simulink model "evaporator_test"  (R2019a)
settings: Solver=VariableStepAuto  StartTime=0.0  StopTime=5000*4  RelTol=1e-3
settings Model: Creator=amah2  LastModifiedBy=kovim

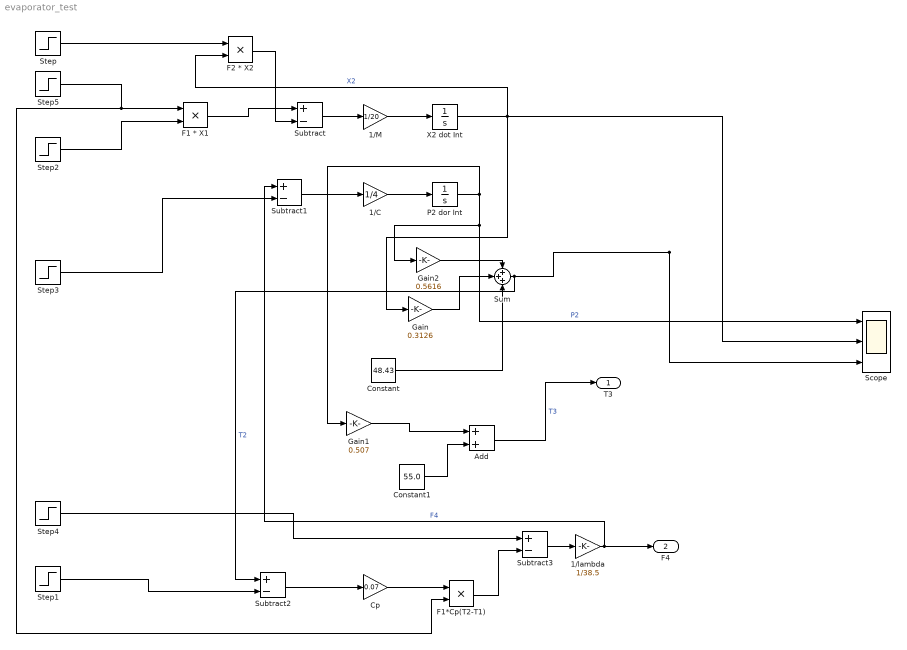
== system evaporator_test ==
  1/C : Gain  Gain=1/4
  1/M : Gain  Gain=1/20
  1/lambda : Gain  Gain=1/38.5
  Add : Sum
  Constant : Constant  Value=48.43
  Constant1 : Constant  Value=55.0
  Cp : Gain  Gain=0.07
  F1 * X1 : Product
  F1*Cp(T2-T1) : Product
  F2 * X2 : Product
  Gain : Gain  Gain=0.3126
  Gain1 : Gain  Gain=0.507
  Gain2 : Gain  Gain=0.5616
  P2 dor Int : Integrator  InitialCondition=50.5
  Scope : Scope  NumInputPorts=3
  Step{,1..5} (6 alike) : Step  SampleTime=0
  Subtract{,1..3} (4 alike) : Sum  Inputs=+-
  Sum : Sum  Inputs=+++
  X2 dot Int : Integrator  InitialCondition=25.0
  "T3 " : Outport
  "F4 " : Outport  Port=2
  wires:
  X2 dot Int/1 -> Scope/2, Gain/1, F2 * X2/2  "X2"
  1/M/1 -> X2 dot Int/1
  Step5/1 -> F1 * X1/1, F1*Cp(T2-T1)/2
  Step2/1 -> F1 * X1/2
  Subtract/1 -> 1/M/1
  F1 * X1/1 -> Subtract/1
  Step/1 -> F2 * X2/1
  F2 * X2/1 -> Subtract/2
  1/C/1 -> P2 dor Int/1
  Subtract1/1 -> 1/C/1
  Step3/1 -> Subtract1/2
  P2 dor Int/1 -> Scope/1, Gain2/1, Gain1/1  "P2"
  Sum/1 -> Subtract2/1, Scope/3  "T2"
  Gain2/1 -> Sum/1
  Gain/1 -> Sum/2
  Constant/1 -> Sum/3
  Constant1/1 -> Add/2
  Gain1/1 -> Add/1
  Add/1 -> "T3 "/1  "T3"
  Subtract3/1 -> 1/lambda/1
  1/lambda/1 -> Subtract1/1, "F4 "/1  "F4"
  Step4/1 -> Subtract3/1
  F1*Cp(T2-T1)/1 -> Subtract3/2
  Cp/1 -> F1*Cp(T2-T1)/1
  Subtract2/1 -> Cp/1
  Step1/1 -> Subtract2/2
